simulink model "plant1srfaa"  (R2019b)
settings: Solver=VariableStepAuto  StartTime=0.0  StopTime=100.0  RelTol=1e-3
libraries: neural x102, cstblocks x1
(part 4 of 4)

== system plant1srfaa/Feed-Forward Neural Network1/Layer 3/Delays 1 ==
  "p{3}" : Inport  PortDimensions=20
      mask Display: e = 0.06;c1 = [120 230 180]/255;c2 = ([120 230 180]+0)/(256+128);c3 = ([120 230 180]+128)/(256+128);patch([0 1 1 0],[0 0 1 1],c1);patch([0 1 1 1-e 1-e 0+e],[0 0 1 1-e 0+e 0+e],c2);patch([0 0 1 1-e 0+e 0+e],[0 1 1 1-e 1-e 0+e],c3);plot([0 1 1 0 0],[0 0 1 1 0]);
  mux : Mux  Inputs=1
      mask Display: e = 0.06;c1 = [120 150 230]/255;c2 = ([120 150 230]+0)/383;c3 = ([120 150 230]+128)/383;patch([0 1 1 0],[0 0 1 1],c1);patch([0 1 1 1-e 1-e 0+e],[0 0 1 1-e 0+e 0+e],c2);patch([0 0 1 1-e 0+e 0+e],[0 1 1 1-e 1-e 0+e],c3);plot([0 1 1 0 0],[0 0 1 1 0]);disp('Mux')
  "pd{3,2}" : Outport
      mask Display: e = 0.06;c1 = [120 230 180]/255;c2 = ([120 230 180]+0)/(256+128);c3 = ([120 230 180]+128)/(256+128);patch([0 1 1 0],[0 0 1 1],c1);patch([0 1 1 1-e 1-e 0+e],[0 0 1 1-e 0+e 0+e],c2);patch([0 0 1 1-e 0+e 0+e],[0 1 1 1-e 1-e 0+e],c3);plot([0 1 1 0 0],[0 0 1 1 0]);
  wires:
  "p{3}"/1 -> mux/1
  mux/1 -> "pd{3,2}"/1

== system plant1srfaa/Feed-Forward Neural Network1/Layer 3/LW{3,2} ==
  "ad{3,2}" : Inport  PortDimensions=20
      mask Display: e = 0.06;c1 = [120 230 180]/255;c2 = ([120 230 180]+0)/(256+128);c3 = ([120 230 180]+128)/(256+128);patch([0 1 1 0],[0 0 1 1],c1);patch([0 1 1 1-e 1-e 0+e],[0 0 1 1-e 0+e 0+e],c2);patch([0 0 1 1-e 0+e 0+e],[0 1 1 1-e 1-e 0+e],c3);plot([0 1 1 0 0],[0 0 1 1 0]);
  "IW{3,2}(1,:)'" : Constant  Value=[0.6077716036230478291457757222815416753292083740234375;0.75452164922096975896437243136460892856121063232421875;-0.74036847149208906415651654242537915706634521484375;0.1728032529314456333668914567169849760830402374267578125;1.995282872068556034861330772400833666324615478515625;0.4323586014591047632649178922292776405811309814453125;0.1992763061327891549456836628451128490269184112548828125;-0.2478821128232095161170178698739618994295597076416015625;0.385834099414470887978723112610168755054473876953125;-0.628704772709232084793029571301303803920745849609375;-0.460066018761585981966533154263743199408054351806640625;-0.334052609195857497237369670983753167092800140380859375;-0.69543381652164082407097112081828527152538299560546875;-0.75762324917207812813302325594122521579265594482421875;-0.128277513458796565970487790764309465885162353515625;0.07114381928119560549728106479960842989385128021240234375;-1.4473543151475334322952903676196001470088958740234375;1.9287456961070035266203603896428830921649932861328125;-0.74087534103903329718576742379809729754924774169921875;-0.261156372927977553644041108782403171062469482421875]
      mask Display: e = 0.06;c1 = [120 150 230]/255;c2 = ([120 150 230]+0)/383;c3 = ([120 150 230]+128)/383;patch([0 1 1 0],[0 0 1 1],c1);patch([0 1 1 1-e 1-e 0+e],[0 0 1 1-e 0+e 0+e],c2);patch([0 0 1 1-e 0+e 0+e],[0 1 1 1-e 1-e 0+e],c3);plot([0 1 1 0 0],[0 0 1 1 0]);disp('weights');
  Mux : Mux  Inputs=1
      mask Display: e = 0.06;c1 = [120 150 230]/255;c2 = ([120 150 230]+0)/383;c3 = ([120 150 230]+128)/383;patch([0 1 1 0],[0 0 1 1],c1);patch([0 1 1 1-e 1-e 0+e],[0 0 1 1-e 0+e 0+e],c2);patch([0 0 1 1-e 0+e 0+e],[0 1 1 1-e 1-e 0+e],c3);plot([0 1 1 0 0],[0 0 1 1 0]);disp('Mux');
  dotprod1 : neural/Weight Functions/dotprod
      settings: SourceProductName=Deep Learning Toolbox
  "lz{3,2}" : Outport
      mask Display: e = 0.06;c1 = [120 230 180]/255;c2 = ([120 230 180]+0)/(256+128);c3 = ([120 230 180]+128)/(256+128);patch([0 1 1 0],[0 0 1 1],c1);patch([0 1 1 1-e 1-e 0+e],[0 0 1 1-e 0+e 0+e],c2);patch([0 0 1 1-e 0+e 0+e],[0 1 1 1-e 1-e 0+e],c3);plot([0 1 1 0 0],[0 0 1 1 0]);
  wires:
  "IW{3,2}(1,:)'"/1 -> dotprod1/1
  "ad{3,2}"/1 -> dotprod1/2
  dotprod1/1 -> Mux/1
  Mux/1 -> "lz{3,2}"/1

== matlab function plant1srfaa/input waveform ==
  data: in1 input; y output; te1 input
function y = fcn(in1,te1)
    if te1<=50
        y=in1;
    else
        y=0;
        
    end
end

== matlab function plant1srfaa/MATLAB Function stress relax ==
  data: e0 input; y output; e1 input; e2 input; te input; ke input
function y = fcn(e0,e1,e2,te,ke)
    k1=818.395;%(2.0286*(e^6));%N/mm
    ne=4559.375;%1.5295*(e^8);
    %if (e0==e1||e1==e2||e2==e0)
     if   (e1>=e0*0.95||e2>=e1*0.95||e0>=e2*0.95||e1<e0*0.95||e2<e1*0.95||e0<e2*0.95)
        %dena=k1*exp(-(te*k1)/ne);
        %dena=k1*(1-exp(-(te*k1)/ne));
        %strress=e0*(ke+dena);
        strress=(e0*ke+e0*(1-k1*exp(-te*(k1/ne))));
     else
        strress=(e0*ke+e0*k1*(exp(-te*(k1/ne))));
        %strress=0;
     end  
     if (strress<0)
       strress=-strress;
     end    
y = strress;
